simulink model "model_p3"  (R2020b)
settings: Solver=FixedStepDiscrete  StartTime=0.0  StopTime=10.0  FixedStep=0.0002  RelTol=1e-3
undefined symbols (not defined in the file): w
settings Model: Creator=ADMIN  LastModifiedBy=ADMIN
settings DataIOCC: ExternalInput=[t, stin]  SaveFormat=Array

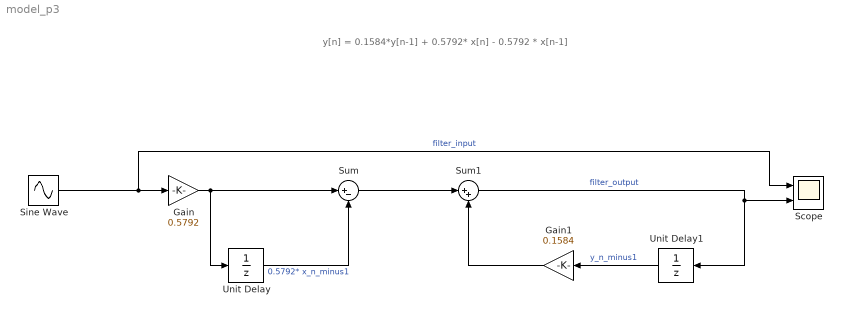
== system model_p3 ==
  note: y[n] = 0.1584*y[n-1] + 0.5792* x[n] - 0.5792 * x[n-1]
  Gain : Gain  Gain=0.5792
  Gain1 : Gain  Gain=0.1584
  Scope : Scope  NumInputPorts=2
  Sine Wave : Sin  Frequency=w  SampleTime=0
  Sum : Sum  Inputs=|+-
  Sum1 : Sum  Inputs=|++
  Unit Delay : UnitDelay  SampleTime=-1  HasFrameUpgradeWarning=on
  Unit Delay1 : UnitDelay  SampleTime=-1  HasFrameUpgradeWarning=on
  wires:
  Gain/1 -> Sum/1, Unit Delay/1
  Unit Delay/1 -> Sum/2  "0.5792* x_n_minus1"
  Sum/1 -> Sum1/1
  Sum1/1 -> Scope/2, Unit Delay1/1  "filter_output"
  Unit Delay1/1 -> Gain1/1  "y_n_minus1"
  Gain1/1 -> Sum1/2
  Sine Wave/1 -> Scope/1, Gain/1  "filter_input"
